simulink model "xuanzhuanzhoufangzhen"  (R2012b)
settings: Solver=ode3  StartTime=0.0  StopTime=20  FixedStep=0.005  RelTol=1e-3
settings Model: Creator=Administrator  LastModifiedBy=Administrator

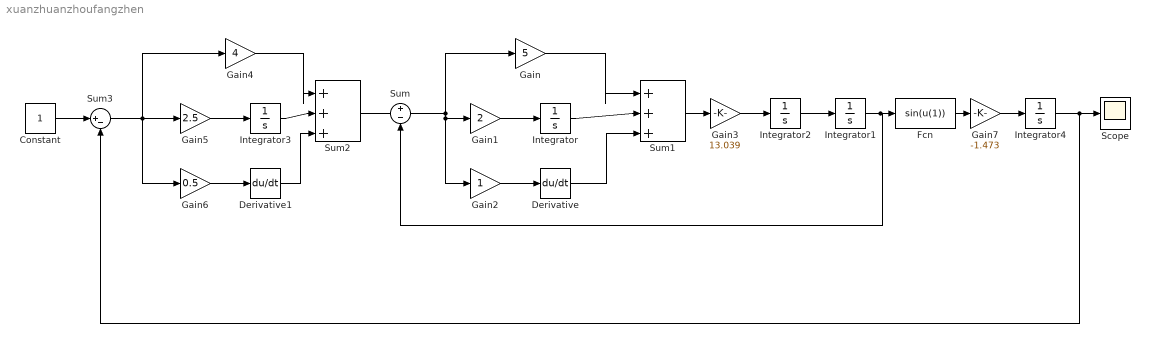
== system xuanzhuanzhoufangzhen ==
  Constant : Constant
  Derivative : Derivative
  Derivative1 : Derivative
  Fcn : Fcn  Expr=sin(u(1))
  Gain : Gain  Gain=5
  Gain1 : Gain  Gain=2
  Gain2 : Gain
  Gain3 : Gain  Gain=13.039
  Gain4 : Gain  Gain=4
  Gain5 : Gain  Gain=2.5
  Gain6 : Gain  Gain=0.5
  Gain7 : Gain  Gain=-1.473
  Integrator{,1..4} (5 alike) : Integrator
  Scope : Scope
      settings: MaxDataPoints=5000000
  Sum : Sum  Inputs=+-
  Sum1 : Sum  Inputs=|+++
  Sum2 : Sum  Inputs=|+++
  Sum3 : Sum  Inputs=|+-
  wires:
  Sum/1 -> Gain2/1, Gain1/1, Gain/1
  Gain1/1 -> Integrator/1
  Gain2/1 -> Derivative/1
  Gain/1 -> Sum1/1
  Integrator/1 -> Sum1/2
  Derivative/1 -> Sum1/3
  Sum1/1 -> Gain3/1
  Gain3/1 -> Integrator2/1
  Integrator2/1 -> Integrator1/1
  Integrator1/1 -> Sum/2, Fcn/1
  Gain5/1 -> Integrator3/1
  Gain6/1 -> Derivative1/1
  Gain4/1 -> Sum2/1
  Integrator3/1 -> Sum2/2
  Derivative1/1 -> Sum2/3
  Constant/1 -> Sum3/1
  Sum3/1 -> Gain6/1, Gain5/1, Gain4/1
  Sum2/1 -> Sum/1
  Fcn/1 -> Gain7/1
  Gain7/1 -> Integrator4/1
  Integrator4/1 -> Sum3/2, Scope/1
